simulink library "SubsystemEnabler"  (R2016b)
settings: Solver=VariableStepAuto  StartTime=0.0  StopTime=10.0  RelTol=1e-3
settings Model: Creator=Nathan  LastModifiedBy=MARCH

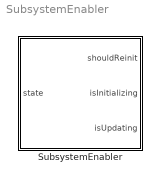
== system SubsystemEnabler ==
  SubsystemEnabler : Subsystem

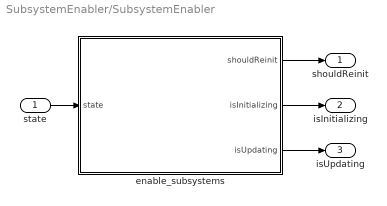
== system SubsystemEnabler/SubsystemEnabler ==
  state : Inport
  enable_subsystems : MATLAB Function  TreatAsAtomicUnit=on
  shouldReinit : Outport
  isInitializing : Outport  Port=2
  isUpdating : Outport  Port=3
  wires:
  state/1 -> enable_subsystems/1(state)
  enable_subsystems/2(isInitializing) -> isInitializing/1
  enable_subsystems/3(isUpdating) -> isUpdating/1
  enable_subsystems/1(shouldReinit) -> shouldReinit/1

== matlab function SubsystemEnabler/enable_subsystems ==
  data: shouldReinit output; state input; isInitializing output; isUpdating output
function [shouldReinit, isInitializing, isUpdating] = enable_subsystems(state)
persistent reinitTimeout;
if(isempty(reinitTimeout))
    reinitTimeout = 0;
end
persistent isInitializingPers;
persistent isUpdatingPers;
persistent shouldReinitPers;
if isempty(isInitializingPers)
    isInitializingPers = false;
    isUpdatingPers = false;
    shouldReinitPers = false;
end
switch state
    case SomanetControlState.startup
        shouldReinitPers = false;
        isInitializingPers = true;
        isUpdatingPers = false;
    case SomanetControlState.tuning
        shouldReinitPers = false;
        isInitializingPers = false;
        isUpdatingPers = true;
    case SomanetControlState.disconnected
        if(reinitTimeout == 0)
            shouldReinitPers = true;
            reinitTimeout = 500;
        else
            shouldReinitPers = false;
            reinitTimeout = reinitTimeout - 1;
        end
        isInitializingPers = false;
        isUpdatingPers = false;
    otherwise
        shouldReinitPers = false;
        isInitializingPers = false;
        isUpdatingPers = false;
end
    isInitializing = isInitializingPers;
    isUpdating = isUpdatingPers;
    shouldReinit = shouldReinitPers;
end
